simulink model "wideband_functest"  (R2019a)
settings: Solver=VariableStepAuto  StartTime=0.0  StopTime=4000  RelTol=1e-3
values from neighbouring files (symbols this model uses):
  shift_schedule = 1023    [pfb_functest_script.m]    (also in wideband_fft_functest_script.m = 0)
undefined symbols (not defined in the file or in its folder): FFT, Wideband_FFT
libraries: xbsIndex_r4 x28, MISC x1
settings Model: Creator=talon  LastModifiedBy=mybur

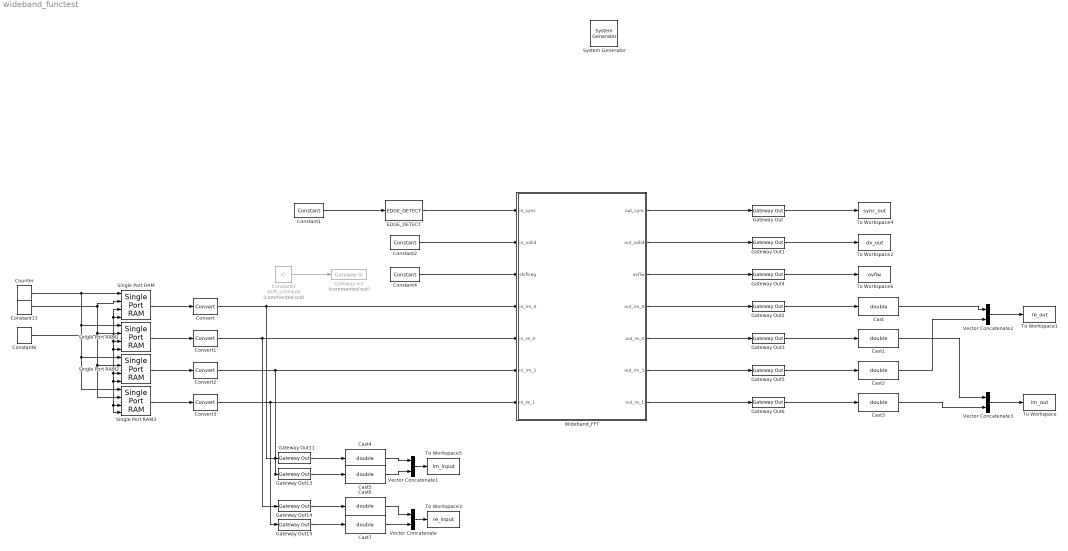
== system wideband_functest ==
  " System Generator" : xbsIndex_r4/ System Generator  Tag=genX  xilinxfamily=kintex7  part=xc7k160t  speed=-2  package=ffg676  synthesis_tool=XST  clock_wrapper=Clock Enables  directory=./netlist  proj_type=Vivado  Synth_file=Vivado Synthesis Defaults  Impl_file=Vivado Implementation Defaults  testbench=off  simulink_period=1  sysclk_period=1000000000  dcm_input_clock_period=10  incr_netlist=off  trim_vbits=Everywhere in SubSystem  dbl_ovrd=According to Block Masks  core_generation=According to Block Masks  run_coregen=off  deprecated_control=off  eval_field=0  block_type=sysgen
  Cast{,1..7} (8 alike) : DataTypeConversion  OutDataTypeStr=double  RndMeth=Nearest
  Constant1 : xbsIndex_r4/Constant  const=1  gui_display_data_type=Boolean  arith_type=Boolean  n_bits=1  bin_pt=0  preci_type=Single  exp_width=8  frac_width=24  explicit_period=on  period=1  equ=P=C  opselect=C  inp2=PCIN>>17  opr=+  inp1=P  carry=CIN  dbl_ovrd=off  block_type=constant
  Constant13 : xbsIndex_r4/Constant  const=0  gui_display_data_type=Fixed-point  arith_type=Signed (2's comp)  n_bits=18  bin_pt=0  preci_type=Single  exp_width=8  frac_width=24  explicit_period=on  period=1  equ=P=C  opselect=C  inp2=PCIN>>17  opr=+  inp1=P  carry=CIN  dbl_ovrd=off  block_type=constant
  Constant2 : xbsIndex_r4/Constant  const=1  gui_display_data_type=Boolean  arith_type=Boolean  n_bits=1  bin_pt=0  preci_type=Single  exp_width=8  frac_width=24  explicit_period=on  period=1  equ=P=C  opselect=C  inp2=PCIN>>17  opr=+  inp1=P  carry=CIN  dbl_ovrd=off  block_type=constant
  Constant3 : Constant  Commented=on  Value=shift_schedule
  Constant4 : xbsIndex_r4/Constant  const=1023  gui_display_data_type=Fixed-point  arith_type=Unsigned  n_bits=10  bin_pt=0  preci_type=Single  exp_width=8  frac_width=24  explicit_period=on  period=1  equ=P=C  opselect=C  inp2=PCIN>>17  opr=+  inp1=P  carry=CIN  dbl_ovrd=off  block_type=constant
  Constant6 : xbsIndex_r4/Constant  const=0  gui_display_data_type=Boolean  arith_type=Boolean  n_bits=16  bin_pt=14  preci_type=Single  exp_width=8  frac_width=24  explicit_period=off  period=1  equ=P=C  opselect=C  inp2=PCIN>>17  opr=+  inp1=P  carry=CIN  dbl_ovrd=off  block_type=constant
  Convert{,1..3} (4 alike) : xbsIndex_r4/Convert  gui_display_data_type=Fixed-point  arith_type="Signed  (2's comp)"  n_bits=input_data_width  bin_pt=0  float_type=Single  exp_bits=8  fraction_bits=24  quantization="Round  (unbiased: Even Values)"  overflow=Wrap  en=off  latency=1  pipeline=off  dbl_ovrd=off  block_type=convert
  Counter : xbsIndex_r4/Counter  cnt_type=Free Running  cnt_to=Inf  operation=Up  start_count=0  cnt_by_val=1  arith_type=Unsigned  n_bits=bram_addr  bin_pt=0  load_pin=off  rst=off  en=off  explicit_period=on  period=1  use_behavioral_HDL=off  implementation=Fabric  dbl_ovrd=off  block_type=counter
  EDGE_DETECT : MISC/EDGE_DETECT  edge_type="\"rising\""  output_pol="\"high\""
      settings: SourceProductName=Casper HDL Blockset
  Gateway In3 : xbsIndex_r4/Gateway In  Commented=on  gui_display_data_type=Fixed-point  arith_type=Unsigned  n_bits=10  bin_pt=0  preci_type=Single  exp_width=8  frac_width=24  rows=1  columns=1  quantization="Round  (unbiased: +/- Inf)"  overflow=Wrap  period=1  UseAsADC=off  ADCChannel='1'  interface=None  automatic_assignment=on  address_offset=hex2dec('00')  intf_name=''  intf_description=''  default_value=0  timing_constraint=None  locs_specified=off  LOCs={}  io_standard={}  inherit_from_input=off  hdl_port=on  dbl_ovrd=off  block_type=gatewayin
  Gateway Out{,2..3,5..6} (5 alike) : xbsIndex_r4/Gateway Out  inherit_from_input=on  hdl_port=on  rows=1  columns=1  UseAsDAC=off  DACChannel='1'  interface=None  automatic_assignment=on  address_offset=hex2dec('00')  intf_name=''  intf_description=''  timing_constraint=None  locs_specified=off  LOCs={}  io_standard={}  block_type=gatewayout
  Gateway Out1 : xbsIndex_r4/Gateway Out  inherit_from_input=off  hdl_port=off  rows=1  columns=1  UseAsDAC=off  DACChannel='1'  interface=None  automatic_assignment=on  address_offset=hex2dec('00')  intf_name=''  intf_description=''  timing_constraint=None  locs_specified=off  LOCs={}  io_standard={}  block_type=gatewayout
  Gateway Out{11,13..15} (4 alike) : xbsIndex_r4/Gateway Out  inherit_from_input=off  hdl_port=on  rows=1  columns=1  UseAsDAC=off  DACChannel='1'  interface=None  automatic_assignment=on  address_offset=hex2dec('00')  intf_name=''  intf_description=''  timing_constraint=None  locs_specified=off  LOCs={}  io_standard={}  block_type=gatewayout
  Gateway Out4 : xbsIndex_r4/Gateway Out  inherit_from_input=off  hdl_port=off  rows=1  columns=1  UseAsDAC=off  DACChannel='1'  interface=None  automatic_assignment=on  address_offset=hex2dec('00')  intf_name=''  intf_description=''  timing_constraint=None  locs_specified=off  LOCs={}  io_standard={}  block_type=gatewayout
  Single Port RAM : xbsIndex_r4/Single Port RAM  depth=bram_depth  initVector=d0  distributed_mem=Block RAM  write_mode=Read After Write  rst=on  init_reg=0  en=off  optimize_latency=off  latency=1  optimize=Area  dbl_ovrd=off  simulation_type=fast_sim  block_type=spram
  Single Port RAM1 : xbsIndex_r4/Single Port RAM  depth=bram_depth  initVector=d1  distributed_mem=Block RAM  write_mode=Read After Write  rst=on  init_reg=0  en=off  optimize_latency=off  latency=1  optimize=Area  dbl_ovrd=off  simulation_type=fast_sim  block_type=spram
  Single Port RAM2 : xbsIndex_r4/Single Port RAM  depth=bram_depth  initVector=d2  distributed_mem=Block RAM  write_mode=Read After Write  rst=on  init_reg=0  en=off  optimize_latency=off  latency=1  optimize=Area  dbl_ovrd=off  simulation_type=fast_sim  block_type=spram
  Single Port RAM3 : xbsIndex_r4/Single Port RAM  depth=bram_depth  initVector=d3  distributed_mem=Block RAM  write_mode=Read After Write  rst=on  init_reg=0  en=off  optimize_latency=off  latency=1  optimize=Area  dbl_ovrd=off  simulation_type=fast_sim  block_type=spram
  To Workspace : ToWorkspace  VariableName=im_out  SaveFormat=Timeseries  SampleTime=-1
  To Workspace1 : ToWorkspace  VariableName=re_out  SaveFormat=Timeseries  SampleTime=-1
  To Workspace2 : ToWorkspace  VariableName=dv_out  SaveFormat=Timeseries  SampleTime=-1
  To Workspace3 : ToWorkspace  VariableName=re_input  SaveFormat=Timeseries  SampleTime=-1
  To Workspace4 : ToWorkspace  VariableName=sync_out  SaveFormat=Timeseries  SampleTime=-1
  To Workspace5 : ToWorkspace  VariableName=im_input  SaveFormat=Timeseries  SampleTime=-1
  To Workspace6 : ToWorkspace  VariableName=ovflw  SaveFormat=Timeseries  SampleTime=-1
  Vector Concatenate{,1..3} (4 alike) : Concatenate  NumInputs=wideband_factor
  Wideband_FFT : Subsystem  AncestorBlock=FFT/Wideband_FFT  mask(Wideband FFT Block){use_separate=on, use_fft_shift=off, use_reorder=on, alt_output=off, wb_factor=2, nof_points=10, in_dat_w=18, twid_dat_w=18, stage_dat_w=18, out_dat_w=18, out_gain_w=0, guard_enable=off, guard_w=2, use_round=1, ovflw_behav="WRAP", pipe_reo_in_place=off, use_dsp="YES", use_variant="4DSP", ram_primitive="block", max_addr_w=8, vendor_technology=Xilinx}
      mask prompts: use_separate "Separate re/im outputs"; use_fft_shift "Reorder frequencies"; use_reorder "Bit reverse output"; alt_output "Alter output data stream"; wb_factor "Wideband factor"; nof_points "Number of points (2^pts)"; in_dat_w "Input data width"; twid_dat_w "FFT twiddle data width"; stage_dat_w "Stage data width"; out_dat_w "Ouput data width"; out_gain_w "Output gain width"; guard_enable "Guard enable"; guard_w "Guard bit width"; use_round "FFT rounding mode: 0-Truncate, 1-Round Even, 2-Round Infinite"; ovflw_behav "Overflow Behaviour"; pipe_reo_in_place "Use single pipelined FFT reorder buffer"; use_dsp "Use DSP for Cmults"; use_variant "Cmult options"; ram_primitive "Ram Primitive"; max_addr_w "Twiddle Max Address Width"; vendor_technology "Vendor"
      mask help: This unit performs an N-Point Wideband FFT on data that is partly applied in serial and partly applied in parallel. This FFT specifically suits applications where the sample clock is higher than the DSP processing clock.
      mask init:
      | Simulink.Block.eval([gcb, '/wb_fft']);
      | 
      | wb_fft_subsys2bb_knit();
      mask Help: https://casper-dspdevel.readthedocs.io/en/latest/wideband_fft.html
      mask Callback use_separate:
      | enab = get_param(gcb,'use_separate');
      | 
      | % Set the 'MaskVisibilities' property for each parameters
      | if strcmp(enab,'on')
      |     set_param(gcb,'use_reorder','on');
      |     set_param(gcb,'use_fft_shift','off');
      |     set_param(gcb,'MaskEnables',{'on','off','off','on','on','on','on','on','on','on','on','on','on','on','on','on','on','on','on','on','on'});
      | else
      |     set_param(gcb,'MaskEnables',{'on','on','on','on','on','on','on','on','on','on','on','on','on','on','on','on','on','on','on','on','on'});
      | end
      mask Callback use_fft_shift:
      | enab = get_param(gcb,'use_fft_shift');
      | 
      | % Set the 'MaskVisibilities' property for each parameters
      | if strcmp(enab,'on')
      |     set_param(gcb,'use_reorder','on');
      |     set_param(gcb,'MaskEnables',{'on','on','off','on','on','on','on','on','on','on','on','on','on','on','on','on','on','on','on','on','on'});
      | else
      |     set_param(gcb,'MaskEnables',{'on','on','on','on','on','on','on','on','on','on','on','on','on','on','on','on','on','on','on','on','on'});
      | end
      mask Callback guard_enable:
      | enab = get_param(gcb,'guard_enable');
      | 
      | % Set the 'MaskVisibilities' property for each parameters
      | if strcmp(enab,'on')
      |     set_param(gcb,'MaskVisibilities',{'on','on','on','on','on','on','on','on','on','on','on','on','on','on','on','on','on','on','on','on','on'});
      | else
      |     set_param(gcb,'MaskVisibilities',{'on','on','on','on','on','on','on','on','on','on','on','on','on','off','on','on','on','on','on','on','on'});
      | end
      mask TypeOptions use_round: 0 | 1 | 2
      mask TypeOptions ovflw_behav: "WRAP" | "SATURATE"
      mask TypeOptions use_dsp: "YES" | "NO"
      mask TypeOptions use_variant: "4DSP" | "3DSP"
      mask TypeOptions ram_primitive: "auto" | "block" | "distributed" | "ultra"
      mask TypeOptions vendor_technology: Xilinx | UniBoard
      mask DialogControl fft_params Prompt: FFT Parameters
      mask DialogControl fft Prompt: FFT
      mask DialogControl data_params Prompt: Data Parameters
      mask DialogControl synth_imp Prompt: FPGA Synth/Imp
  wires:
  Constant1/1 -> EDGE_DETECT/1
  Wideband_FFT/3(ovflw) -> Gateway Out4/1
  Gateway Out2/1 -> Cast/1
  Wideband_FFT/1(out_sync) -> Gateway Out/1
  Vector Concatenate/1 -> To Workspace3/1
  Vector Concatenate1/1 -> To Workspace5/1
  Vector Concatenate2/1 -> To Workspace1/1
  Vector Concatenate3/1 -> To Workspace/1
  Constant6/1 -> Single Port RAM/3, Single Port RAM/4, Single Port RAM3/4, Single Port RAM3/3, Single Port RAM2/4, Single Port RAM2/3, Single Port RAM1/4, Single Port RAM1/3
  Constant3/1 -> Gateway In3/1
  Counter/1 -> Single Port RAM3/1, Single Port RAM2/1, Single Port RAM1/1, Single Port RAM/1
  Constant13/1 -> Single Port RAM/2, Single Port RAM3/2, Single Port RAM2/2, Single Port RAM1/2
  Single Port RAM3/1 -> Convert3/1
  Single Port RAM2/1 -> Convert2/1
  Single Port RAM1/1 -> Convert1/1
  Single Port RAM/1 -> Convert/1
  Gateway Out11/1 -> Cast4/1
  Gateway Out13/1 -> Cast5/1
  Gateway Out14/1 -> Cast6/1
  Gateway Out15/1 -> Cast7/1
  Cast/1 -> Vector Concatenate2/1
  Gateway Out3/1 -> Cast1/1
  Cast1/1 -> Vector Concatenate3/1
  Gateway Out5/1 -> Cast2/1
  Cast2/1 -> Vector Concatenate2/2
  Gateway Out6/1 -> Cast3/1
  Cast3/1 -> Vector Concatenate3/2
  Cast4/1 -> Vector Concatenate1/1
  Cast5/1 -> Vector Concatenate1/2
  Cast6/1 -> Vector Concatenate/1
  Cast7/1 -> Vector Concatenate/2
  Convert/1 -> Wideband_FFT/4(in_im_0), Gateway Out11/1
  Convert1/1 -> Gateway Out14/1, Wideband_FFT/5(in_re_0)
  Convert2/1 -> Wideband_FFT/6(in_im_1), Gateway Out13/1
  Convert3/1 -> Gateway Out15/1, Wideband_FFT/7(in_re_1)
  Wideband_FFT/5(out_re_0) -> Gateway Out3/1
  Wideband_FFT/6(out_im_1) -> Gateway Out5/1
  Wideband_FFT/7(out_re_1) -> Gateway Out6/1
  Gateway Out4/1 -> To Workspace6/1
  Constant4/1 -> Wideband_FFT/3(shiftreg)
  Constant2/1 -> Wideband_FFT/2(in_valid)
  Wideband_FFT/4(out_im_0) -> Gateway Out2/1
  Wideband_FFT/2(out_valid) -> Gateway Out1/1
  EDGE_DETECT/1 -> Wideband_FFT/1(in_sync)
  Gateway Out/1 -> To Workspace4/1
  Gateway Out1/1 -> To Workspace2/1

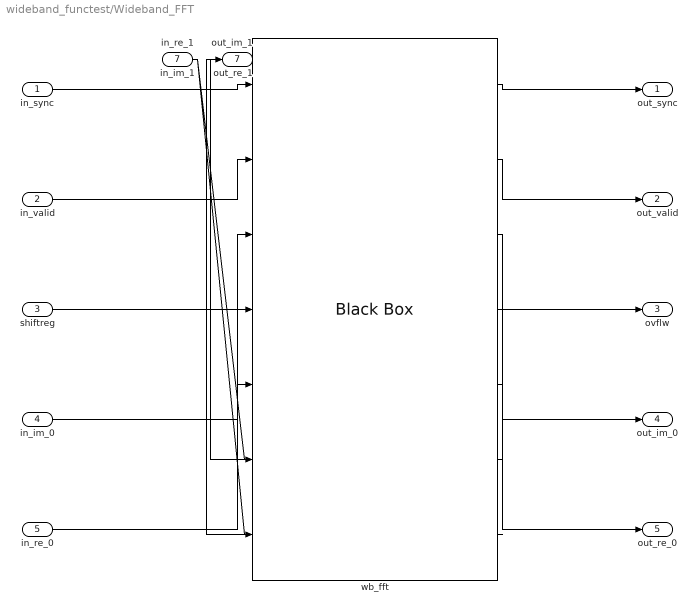
== system wideband_functest/Wideband_FFT ==
  in_sync : Inport
  in_valid : Inport  Port=2
  shiftreg : Inport  Port=3
  in_im_0 : Inport  Port=4
  in_re_0 : Inport  Port=5
  in_im_1 : Inport  Port=6
  in_re_1 : Inport  Port=7
  wb_fft : xbsIndex_r4/Black Box  init_code=casper_wb_fft_config  sim_method=ISE Simulator  verbose=off  block_type=blackbox2
  out_sync : Outport
  out_valid : Outport  Port=2
  ovflw : Outport  Port=3
  out_im_0 : Outport  Port=4
  out_re_0 : Outport  Port=5
  out_im_1 : Outport  Port=6
  out_re_1 : Outport  Port=7
  wires:
  wb_fft/1 -> out_sync/1
  wb_fft/2 -> out_valid/1
  wb_fft/3 -> ovflw/1
  wb_fft/4 -> out_im_0/1
  wb_fft/5 -> out_re_0/1
  in_sync/1 -> wb_fft/1
  in_valid/1 -> wb_fft/2
  shiftreg/1 -> wb_fft/3
  in_im_0/1 -> wb_fft/4
  in_re_0/1 -> wb_fft/5
  in_im_1/1 -> wb_fft/6
  in_re_1/1 -> wb_fft/7
  wb_fft/6 -> out_im_1/1
  wb_fft/7 -> out_re_1/1
